simulink model "Yaw_Diff_CS9_Lab"  (R2020a)
settings: Solver=ode45  StartTime=0  StopTime=10  FixedStep=0.002  RelTol=1e-3  AbsTol=1e-6
libraries: simulink x4, simulink_extras x2, Solver_SF x1
settings Model: ExtModeTrigMode=oneshot  ExtModeArmWhenConnect=off  Creator=ywata  LastModifiedBy=S288668
settings SolverCC: AutoScaleAbsTol=off
settings DataIOCC: SaveFormat=Array  SignalLoggingSaveFormat=ModelDataLogs  ReturnWorkspaceOutputs=off  SignalLoggingName=sigsOut
settings OptimizationCC: BooleanDataType=off  ExpressionDepthLimit=2147483647  LifeSpan=inf
settings DebuggingCC: SaveWithParameterizedLinksMsg=none  UnderspecifiedInitializationDetection=Classic  MergeDetectMultiDrivingBlocksExec=none  SignalResolutionControl=TryResolveAllWithWarning  MultiTaskDSMMsg=warning  MultiTaskCondExecSysMsg=none  FcnCallInpInsideContextMsg=warning  StateNameClashWarn=warning  SFUnexpectedBacktrackingDiag=warning  SFNoUnconditionalDefaultTransitionDiag=warning  SFExecutionAtInitializationDiag=none  ArithmeticOperatorsInVariantConditions=warning
settings HardwareCC: ProdBitPerPointer=32  ProdBitPerSizeT=32  ProdBitPerPtrDiffT=32  ProdLargestAtomicFloat=None  ProdIntDivRoundTo=Undefined  ProdEndianess=Unspecified  ProdWordSize=32  ProdHWDeviceType=32-bit Generic  TargetUnknown=on
settings ModelReferenceCC: PropagateSignalLabelsOutOfModel=off
settings SFSimCC: SimUseLocalCustomCode=off  CustomCodeUndefinedFunction=UseInterfaceOnly
settings RTWCC: TemplateMakefile=grt_vc.tmf  RTWUseLocalCustomCode=off
settings CodeAppCC: StateflowObjectComments=on
settings GRTTargetCC: TargetLangStandard=C89/C90 (ANSI)  CombineOutputUpdateFcns=off  GRTInterface=on
settings ConfigComp: CovMetricSettings=dw  CovHtmlReporting=on  CovSaveCumulativeToWorkspaceVar=on  CovSaveSingleToWorkspaceVar=on  CovExternalEMLEnable=off

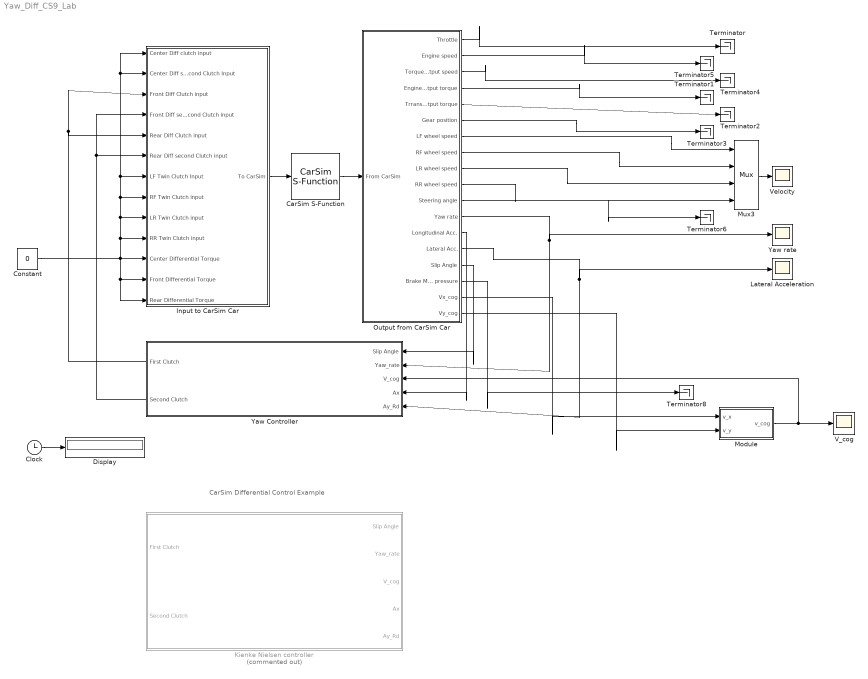
== system Yaw_Diff_CS9_Lab ==
  note: CarSim Differential Control Example
  CarSim S-Function : Solver_SF/CarSim S-Function  Priority=1  SIMFILE=simfile.sim
  Clock : Clock
  Constant : Constant  Value=0
  Display : Display
      settings: Format=bank  Decimation=100
  Input to CarSim Car : Subsystem
  Kienke Nielsen controller : Subsystem  Commented=on
  Lateral Acceleration : Scope
  Module : Subsystem
  Mux3 : Mux
  Output from CarSim Car : Subsystem
  Terminator{,1..6,8} (8 alike) : Terminator
  V_cog : Scope
  Velocity : Scope
  Yaw Controller : Subsystem  mask{YAW=0.06, CONTROL=0.72}
      mask prompts: YAW "Yaw Control Gain (-)"; CONTROL "Control Gain (-)"
  Yaw rate : Scope
  wires:
  Constant/1 -> Input to CarSim Car/11(Center Differential Torque), Input to CarSim Car/12("Front Differential Torque "), Input to CarSim Car/13(Rear Differential Torque), Input to CarSim Car/8(RF Twin Clutch input), Input to CarSim Car/7(LF Twin Clutch Input), Input to CarSim Car/2(Center Diff second Clutch Input), Input to CarSim Car/1(Center Diff clutch input), Input to CarSim Car/9(LR Twin Clutch input), Input to CarSim Car/10(RR Twin Clutch input)
  CarSim S-Function/1 -> Output from CarSim Car/1(From CarSim)
  Input to CarSim Car/1(To CarSim) -> CarSim S-Function/1
  Yaw Controller/1(First Clutch) -> Input to CarSim Car/3(Front Diff Clutch input), Input to CarSim Car/5(Rear Diff Clutch input)
  Yaw Controller/2(Second Clutch) -> Input to CarSim Car/4(Front Diff second Clutch input), Input to CarSim Car/6(Rear Diff second Clutch input)
  Clock/1 -> Display/1
  Mux3/1 -> Velocity/1
  Output from CarSim Car/7(LF wheel speed) -> Mux3/1
  Output from CarSim Car/8(RF wheel speed) -> Mux3/2
  Output from CarSim Car/9(LR wheel speed) -> Mux3/3
  Output from CarSim Car/10(RR wheel speed) -> Mux3/4
  Output from CarSim Car/1(Throttle) -> Terminator/1
  Output from CarSim Car/4(Engine output torque) -> Terminator1/1
  Output from CarSim Car/5(Trransmission output torque) -> Terminator2/1
  Output from CarSim Car/6(Gear position) -> Terminator3/1
  Output from CarSim Car/3(Torque converter output speed) -> Terminator4/1
  Output from CarSim Car/2(Engine speed) -> Terminator5/1
  Output from CarSim Car/11(Steering angle) -> Terminator6/1
  Output from CarSim Car/13(Longitudinal Acc.) -> Yaw Controller/4(Ax)
  Output from CarSim Car/16(Brake M/C pressure) -> Terminator8/1
  Output from CarSim Car/14(Lateral Acc.) -> Yaw Controller/5(Ay_Rd), Lateral Acceleration/1
  Output from CarSim Car/15(Slip Angle) -> Yaw Controller/1(Slip Angle)
  Output from CarSim Car/12(Yaw rate) -> Yaw Controller/2(Yaw_rate), Yaw rate/1
  Output from CarSim Car/17(Vx_cog) -> Module/1(v_x)
  Output from CarSim Car/18(Vy_cog) -> Module/2(v_y)
  Module/1(v_cog) -> V_cog/1, Yaw Controller/3(V_cog)

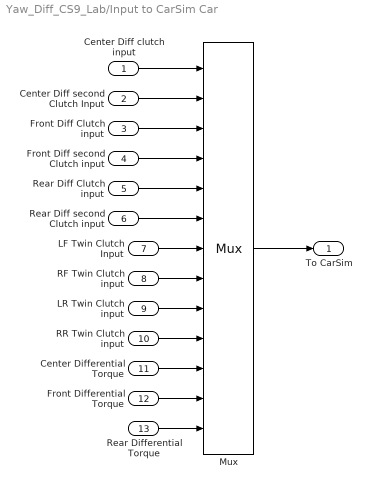
== system Yaw_Diff_CS9_Lab/Input to CarSim Car ==
  Center Diff clutch input : Inport
  Center Diff second Clutch Input : Inport  Port=2
  Front Diff Clutch input : Inport  Port=3
  Front Diff second Clutch input : Inport  Port=4
  Rear Diff Clutch input : Inport  Port=5
  Rear Diff second Clutch input : Inport  Port=6
  LF Twin Clutch Input : Inport  Port=7
  RF Twin Clutch input : Inport  Port=8
  LR Twin Clutch input : Inport  Port=9
  RR Twin Clutch input : Inport  Port=10
  Center Differential Torque : Inport  Port=11
  "Front Differential Torque " : Inport  Port=12
  Rear Differential Torque : Inport  Port=13
  Mux : Mux  Inputs=13
  To CarSim : Outport
  wires:
  Mux/1 -> To CarSim/1
  Center Differential Torque/1 -> Mux/11
  Rear Differential Torque/1 -> Mux/13
  "Front Differential Torque "/1 -> Mux/12
  RR Twin Clutch input/1 -> Mux/10
  LR Twin Clutch input/1 -> Mux/9
  RF Twin Clutch input/1 -> Mux/8
  LF Twin Clutch Input/1 -> Mux/7
  Rear Diff second Clutch input/1 -> Mux/6
  Rear Diff Clutch input/1 -> Mux/5
  Front Diff second Clutch input/1 -> Mux/4
  Front Diff Clutch input/1 -> Mux/3
  Center Diff second Clutch Input/1 -> Mux/2
  Center Diff clutch input/1 -> Mux/1

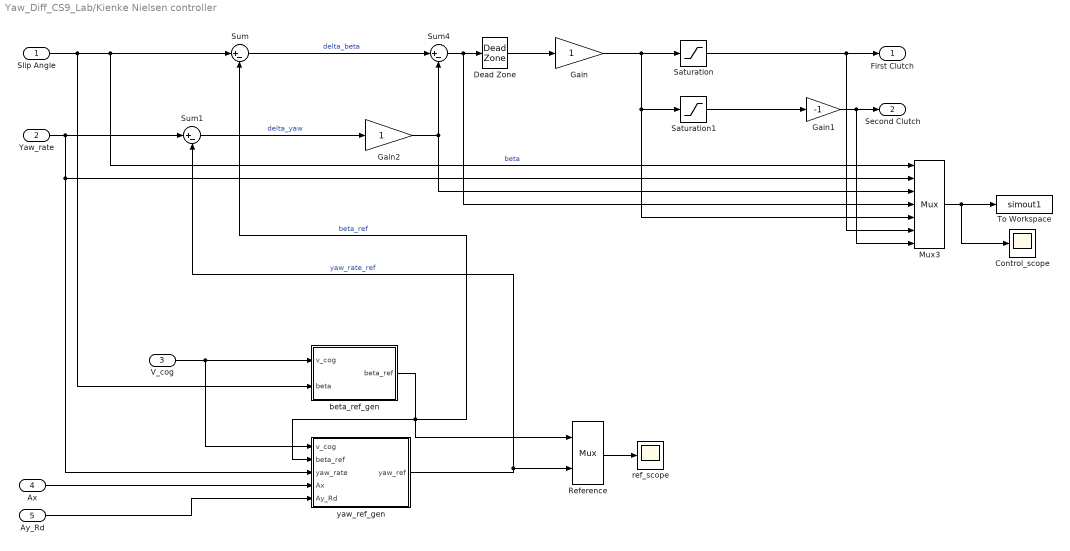
== system Yaw_Diff_CS9_Lab/Kienke Nielsen controller ==
  Slip Angle : Inport
  Yaw_rate : Inport  Port=2
  V_cog : Inport  Port=3
  Ax : Inport  Port=4
  Ay_Rd : Inport  Port=5
  Control_scope : Scope
  Dead Zone : DeadZone  SaturateOnIntegerOverflow=on
  Gain : Gain
  Gain1 : Gain  Gain=-1  SaturateOnIntegerOverflow=on  OutDataTypeStr=Inherit: Same as input  ParamDataTypeStr=Inherit: Same as input
  Gain2 : Gain
  Mux3 : Mux  Inputs=7
  Reference : Mux  Inputs=2
  Saturation : Saturate  UpperLimit=1  LowerLimit=0
  Saturation1 : Saturate  UpperLimit=0  LowerLimit=-1
  Sum : Sum  Inputs=|+-
  Sum1 : Sum  Inputs=|+-
  Sum4 : Sum  Inputs=|+-  InputSameDT=on  SaturateOnIntegerOverflow=on  OutDataTypeStr=Inherit: Same as first input
  To Workspace : ToWorkspace  VariableName=simout1  SaveFormat=Timeseries  SampleTime=-1
  beta_ref_gen : Subsystem
  ref_scope : Scope
  yaw_ref_gen : Subsystem
  First Clutch : Outport
  Second Clutch : Outport  Port=2
  wires:
  yaw_ref_gen/1(yaw_ref) -> Sum1/2, Reference/2  "yaw_rate_ref"
  Ay_Rd/1 -> yaw_ref_gen/5(Ay_Rd)
  Gain1/1 -> Mux3/7, Second Clutch/1
  Mux3/1 -> To Workspace/1, Control_scope/1
  V_cog/1 -> yaw_ref_gen/1(v_cog), beta_ref_gen/1(v_cog)
  Saturation/1 -> Mux3/6, First Clutch/1
  beta_ref_gen/1(beta_ref) -> yaw_ref_gen/2(beta_ref), Sum/2, Reference/1  "beta_ref"
  Slip Angle/1 -> Sum/1, Mux3/1, beta_ref_gen/2(beta)  "beta"
  Sum4/1 -> Mux3/4, Dead Zone/1
  Reference/1 -> ref_scope/1
  Ax/1 -> yaw_ref_gen/4(Ax)
  Yaw_rate/1 -> Sum1/1, yaw_ref_gen/3(yaw_rate), Mux3/2
  Saturation1/1 -> Gain1/1
  Gain/1 -> Saturation/1, Mux3/5, Saturation1/1
  Dead Zone/1 -> Gain/1
  Gain2/1 -> Mux3/3, Sum4/2
  Sum/1 -> Sum4/1  "delta_beta"
  Sum1/1 -> Gain2/1  "delta_yaw"

== system Yaw_Diff_CS9_Lab/Module ==
  v_x : Inport
  v_y : Inport  Port=2
  Sqrt : Sqrt  SaturateOnIntegerOverflow=on
  Square : Math  Operator=square  SaturateOnIntegerOverflow=on
  Square1 : Math  Operator=square  SaturateOnIntegerOverflow=on
  Sum : Sum  Inputs=|++
  v_cog : Outport
  wires:
  v_x/1 -> Square/1
  v_y/1 -> Square1/1
  Square/1 -> Sum/1
  Square1/1 -> Sum/2
  Sum/1 -> Sqrt/1
  Sqrt/1 -> v_cog/1

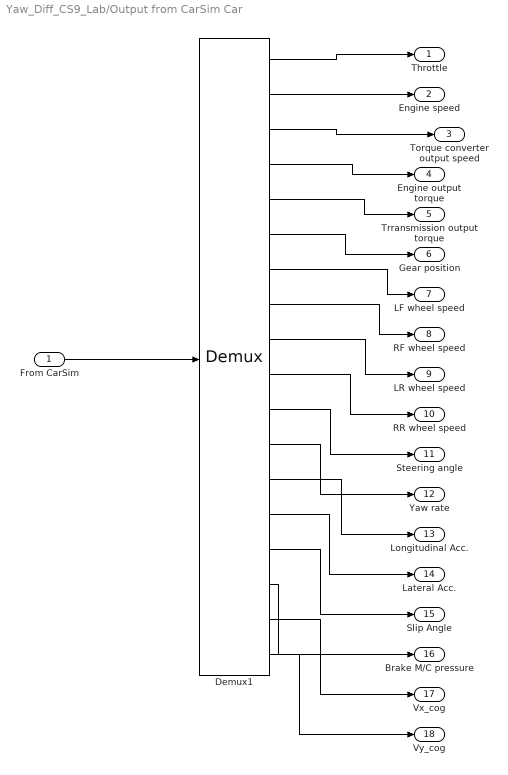
== system Yaw_Diff_CS9_Lab/Output from CarSim Car ==
  From CarSim : Inport
  Demux1 : Demux  Outputs=18
      settings: DisplayOption=none
  Throttle : Outport
  Engine speed : Outport  Port=2
  Torque converter output speed : Outport  Port=3
  Engine output torque : Outport  Port=4
  Trransmission output torque : Outport  Port=5
  Gear position : Outport  Port=6
  LF wheel speed : Outport  Port=7
  RF wheel speed : Outport  Port=8
  LR wheel speed : Outport  Port=9
  RR wheel speed : Outport  Port=10
  Steering angle : Outport  Port=11
  Yaw rate : Outport  Port=12
  Longitudinal Acc. : Outport  Port=13
  Lateral Acc. : Outport  Port=14
  Slip Angle : Outport  Port=15
  Brake M/C pressure : Outport  Port=16
  Vx_cog : Outport  Port=17
  Vy_cog : Outport  Port=18
  wires:
  From CarSim/1 -> Demux1/1
  Demux1/1 -> Throttle/1
  Demux1/2 -> Engine speed/1
  Demux1/3 -> Torque converter output speed/1
  Demux1/7 -> LF wheel speed/1
  Demux1/13 -> Longitudinal Acc./1
  Demux1/14 -> Lateral Acc./1
  Demux1/8 -> RF wheel speed/1
  Demux1/9 -> LR wheel speed/1
  Demux1/10 -> RR wheel speed/1
  Demux1/11 -> Steering angle/1
  Demux1/12 -> Yaw rate/1
  Demux1/4 -> Engine output torque/1
  Demux1/5 -> Trransmission output torque/1
  Demux1/6 -> Gear position/1
  Demux1/15 -> Slip Angle/1
  Demux1/16 -> Brake M/C pressure/1
  Demux1/17 -> Vx_cog/1
  Demux1/18 -> Vy_cog/1

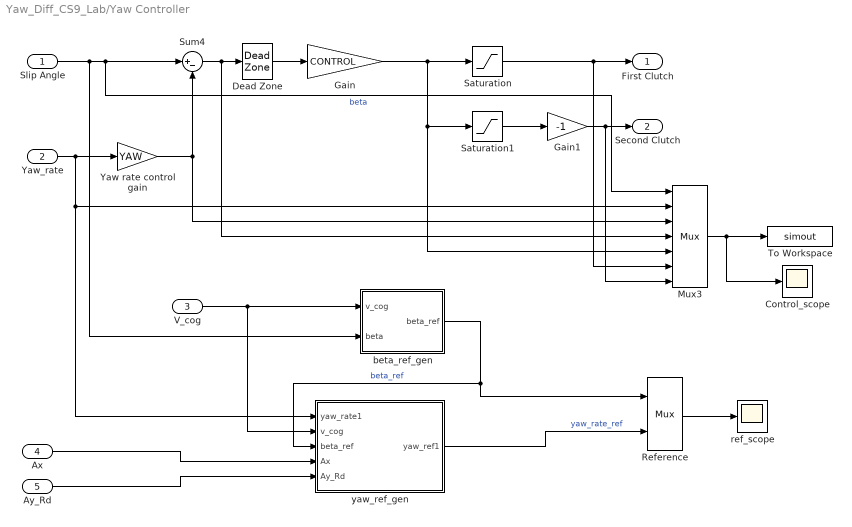
== system Yaw_Diff_CS9_Lab/Yaw Controller ==
  Slip Angle : Inport
  Yaw_rate : Inport  Port=2
  V_cog : Inport  Port=3
  Ax : Inport  Port=4
  Ay_Rd : Inport  Port=5
  Control_scope : Scope
  Dead Zone : DeadZone  SaturateOnIntegerOverflow=on
  Gain : Gain  Gain=CONTROL  SaturateOnIntegerOverflow=on  OutDataTypeStr=Inherit: Same as input  ParamDataTypeStr=Inherit: Same as input
  Gain1 : Gain  Gain=-1  SaturateOnIntegerOverflow=on  OutDataTypeStr=Inherit: Same as input  ParamDataTypeStr=Inherit: Same as input
  Mux3 : Mux  Inputs=7
  Reference : Mux  Inputs=2
  Saturation : Saturate  UpperLimit=1  LowerLimit=0
  Saturation1 : Saturate  UpperLimit=0  LowerLimit=-1
  Sum4 : Sum  Inputs=|+-  InputSameDT=on  SaturateOnIntegerOverflow=on  OutDataTypeStr=Inherit: Same as first input
  To Workspace : ToWorkspace  VariableName=simout  SaveFormat=Timeseries  SampleTime=-1
  Yaw rate control gain : Gain  Gain=YAW  SaturateOnIntegerOverflow=on  OutDataTypeStr=Inherit: Same as input  ParamDataTypeStr=Inherit: Same as input
  beta_ref_gen : Subsystem
  ref_scope : Scope
  yaw_ref_gen : Subsystem
  First Clutch : Outport
  Second Clutch : Outport  Port=2
  wires:
  Yaw rate control gain/1 -> Mux3/3, Sum4/2
  Yaw_rate/1 -> yaw_ref_gen/1(yaw_rate1), Mux3/2, Yaw rate control gain/1
  Dead Zone/1 -> Gain/1
  Sum4/1 -> Mux3/4, Dead Zone/1
  Gain/1 -> Saturation/1, Mux3/5, Saturation1/1
  Saturation1/1 -> Gain1/1
  Saturation/1 -> Mux3/6, First Clutch/1
  Gain1/1 -> Mux3/7, Second Clutch/1
  Slip Angle/1 -> Mux3/1, Sum4/1, beta_ref_gen/2(beta)  "beta"
  Mux3/1 -> To Workspace/1, Control_scope/1
  Reference/1 -> ref_scope/1
  V_cog/1 -> yaw_ref_gen/2(v_cog), beta_ref_gen/1(v_cog)
  beta_ref_gen/1(beta_ref) -> yaw_ref_gen/3(beta_ref), Reference/1  "beta_ref"
  yaw_ref_gen/1(yaw_ref1) -> Reference/2  "yaw_rate_ref"
  Ay_Rd/1 -> yaw_ref_gen/5(Ay_Rd)
  Ax/1 -> yaw_ref_gen/4(Ax)

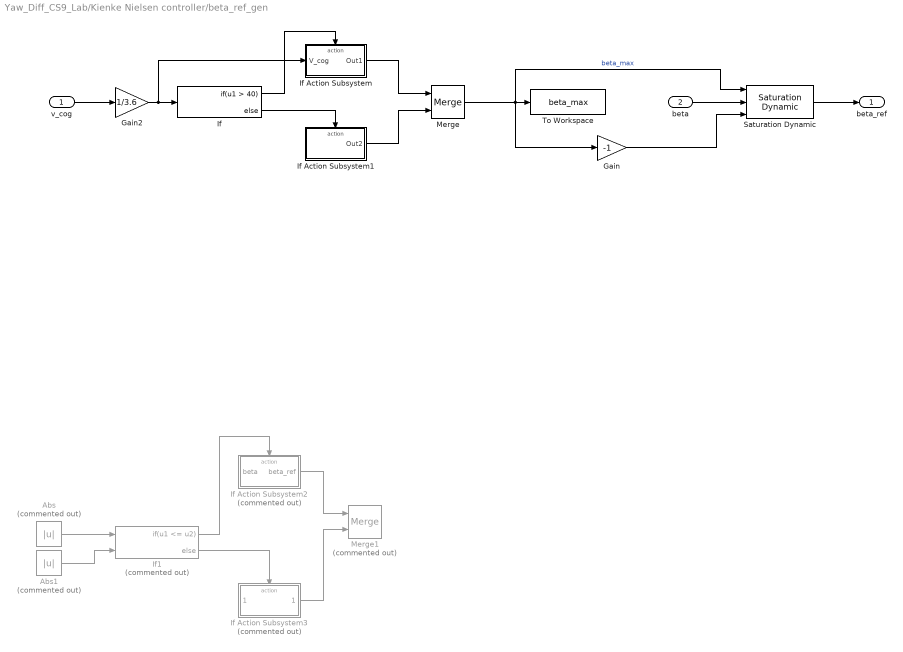
== system Yaw_Diff_CS9_Lab/Kienke Nielsen controller/beta_ref_gen ==
  v_cog : Inport
  beta : Inport  Port=2
  Abs : Abs  Commented=on
  Abs1 : Abs  Commented=on
  Gain : Gain  Gain=-1
  Gain2 : Gain  Gain=1/3.6
  If : If  IfExpression=u1 > 40
  If Action Subsystem : Subsystem  TreatAsAtomicUnit=on
  If Action Subsystem1 : Subsystem  TreatAsAtomicUnit=on
  If Action Subsystem2 : Subsystem  Commented=on  TreatAsAtomicUnit=on
  If Action Subsystem3 : Subsystem  Commented=on  TreatAsAtomicUnit=on
  If1 : If  Commented=on  NumInputs=2  IfExpression=u1 <= u2
  Merge : Merge
  Merge1 : Merge  Commented=on
  Saturation Dynamic : simulink/Discontinuities/Saturation Dynamic  OutMin=[]  OutMax=[]  OutDataTypeStr=Inherit: Same as second input  OutDataType=fixdt(1, 16)  OutScaling=2^-10  DoSatur=off
  To Workspace : ToWorkspace  VariableName=beta_max  SaveFormat=Timeseries  SampleTime=-1
  beta_ref : Outport
  wires:
  If/1 -> If Action Subsystem/Action
  Gain2/1 -> If Action Subsystem/1(V_cog), If/1
  If Action Subsystem/1(Out1) -> Merge/1
  If/2 -> If Action Subsystem1/Action
  If Action Subsystem1/1(Out2) -> Merge/2
  v_cog/1 -> Gain2/1
  Merge/1 -> Gain/1, Saturation Dynamic/1, To Workspace/1  "beta_max"
  Abs1/1 -> If1/2
  ? -> If Action Subsystem2/1(beta), Abs/1
  If1/2 -> If Action Subsystem3/Action
  Abs/1 -> If1/1
  If Action Subsystem3/1(beta_ref) -> Merge1/2
  If Action Subsystem2/1(beta_ref) -> Merge1/1
  ? -> If Action Subsystem3/1(beta_max), Abs1/1  "beta_max"
  If1/1 -> If Action Subsystem2/Action
  Saturation Dynamic/1 -> beta_ref/1
  beta/1 -> Saturation Dynamic/2
  Gain/1 -> Saturation Dynamic/3

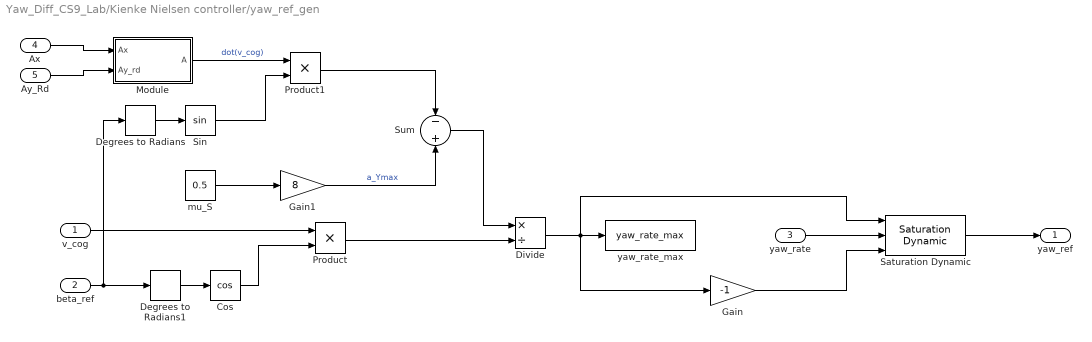
== system Yaw_Diff_CS9_Lab/Kienke Nielsen controller/yaw_ref_gen ==
  v_cog : Inport
  beta_ref : Inport  Port=2
  yaw_rate : Inport  Port=3
  Ax : Inport  Port=4
  Ay_Rd : Inport  Port=5
  Cos : Trigonometry  Operator=cos
  Degrees to Radians : simulink_extras/Transformations/Degrees to Radians
  Degrees to Radians1 : simulink_extras/Transformations/Degrees to Radians
  Divide : Product  Inputs=*/
  Gain : Gain  Gain=-1
  Gain1 : Gain  Gain=8
  Module : Subsystem
  Product : Product
  Product1 : Product
  Saturation Dynamic : simulink/Discontinuities/Saturation Dynamic  OutMin=[]  OutMax=[]  OutDataTypeStr=Inherit: Same as second input  OutDataType=fixdt(1, 16)  OutScaling=2^-10  DoSatur=off
  Sin : Trigonometry
  Sum : Sum  Inputs=-|+
  mu_S : Constant  Value=0.5
  yaw_rate_max : ToWorkspace  VariableName=yaw_rate_max  SaveFormat=Timeseries  SampleTime=-1
  yaw_ref : Outport
  wires:
  beta_ref/1 -> Degrees to Radians/1, Degrees to Radians1/1
  v_cog/1 -> Product/1
  Cos/1 -> Product/2
  Sin/1 -> Product1/2
  Product1/1 -> Sum/1
  Product/1 -> Divide/2
  Sum/1 -> Divide/1
  Divide/1 -> Gain/1, Saturation Dynamic/1, yaw_rate_max/1
  yaw_rate/1 -> Saturation Dynamic/2
  Saturation Dynamic/1 -> yaw_ref/1
  Module/1(A) -> Product1/1  "dot(v_cog)"
  Ax/1 -> Module/1(Ax)
  Ay_Rd/1 -> Module/2(Ay_rd)
  mu_S/1 -> Gain1/1
  Gain1/1 -> Sum/2  "a_Ymax"
  Gain/1 -> Saturation Dynamic/3
  Degrees to Radians/1 -> Sin/1
  Degrees to Radians1/1 -> Cos/1

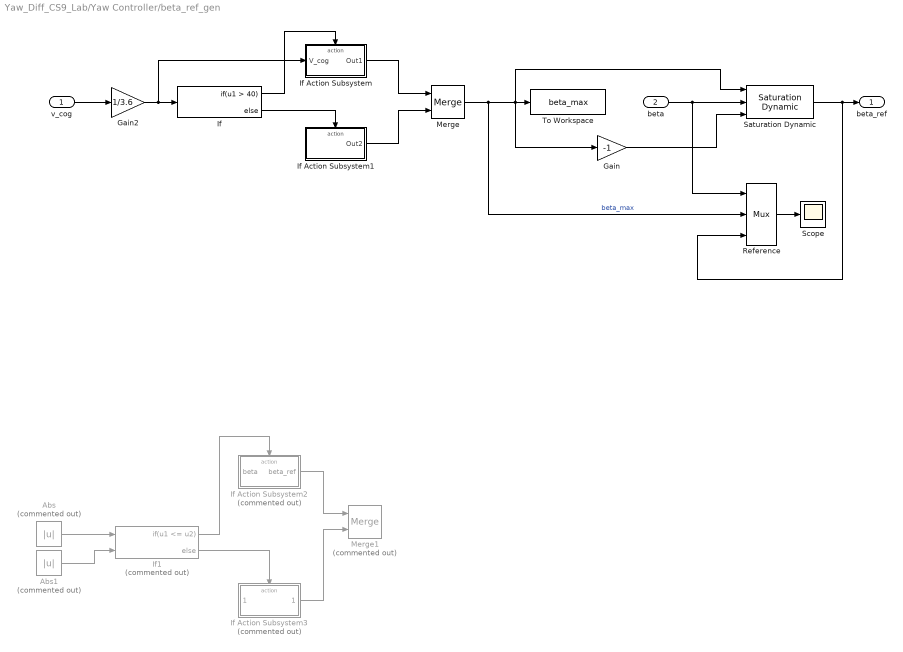
== system Yaw_Diff_CS9_Lab/Yaw Controller/beta_ref_gen ==
  v_cog : Inport
  beta : Inport  Port=2
  Abs : Abs  Commented=on
  Abs1 : Abs  Commented=on
  Gain : Gain  Gain=-1
  Gain2 : Gain  Gain=1/3.6
  If : If  IfExpression=u1 > 40
  If Action Subsystem : Subsystem  TreatAsAtomicUnit=on
  If Action Subsystem1 : Subsystem  TreatAsAtomicUnit=on
  If Action Subsystem2 : Subsystem  Commented=on  TreatAsAtomicUnit=on
  If Action Subsystem3 : Subsystem  Commented=on  TreatAsAtomicUnit=on
  If1 : If  Commented=on  NumInputs=2  IfExpression=u1 <= u2
  Merge : Merge
  Merge1 : Merge  Commented=on
  Reference : Mux  Inputs=3
  Saturation Dynamic : simulink/Discontinuities/Saturation Dynamic  OutMin=[]  OutMax=[]  OutDataTypeStr=Inherit: Same as second input  OutDataType=fixdt(1, 16)  OutScaling=2^-10  DoSatur=off
  Scope : Scope
  To Workspace : ToWorkspace  VariableName=beta_max  SaveFormat=Timeseries  SampleTime=-1
  beta_ref : Outport
  wires:
  If/1 -> If Action Subsystem/Action
  Gain2/1 -> If Action Subsystem/1(V_cog), If/1
  If Action Subsystem/1(Out1) -> Merge/1
  If/2 -> If Action Subsystem1/Action
  If Action Subsystem1/1(Out2) -> Merge/2
  v_cog/1 -> Gain2/1
  Merge/1 -> Reference/2, Gain/1, Saturation Dynamic/1, To Workspace/1  "beta_max"
  Abs1/1 -> If1/2
  ? -> If Action Subsystem2/1(beta), Abs/1
  If1/2 -> If Action Subsystem3/Action
  Abs/1 -> If1/1
  If Action Subsystem3/1(beta_ref) -> Merge1/2
  If Action Subsystem2/1(beta_ref) -> Merge1/1
  ? -> If Action Subsystem3/1(beta_max), Abs1/1  "beta_max"
  If1/1 -> If Action Subsystem2/Action
  Saturation Dynamic/1 -> Reference/3, beta_ref/1
  beta/1 -> Reference/1, Saturation Dynamic/2
  Gain/1 -> Saturation Dynamic/3
  Reference/1 -> Scope/1

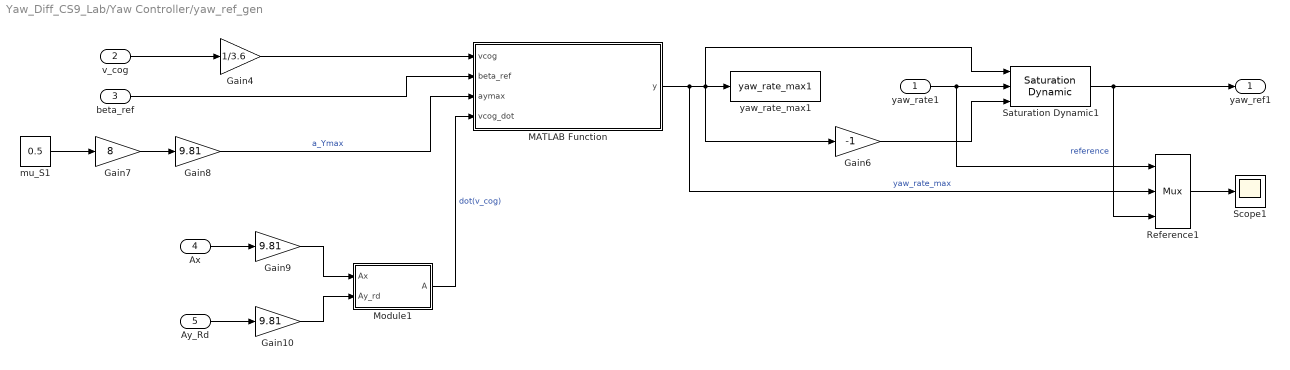
== system Yaw_Diff_CS9_Lab/Yaw Controller/yaw_ref_gen ==
  yaw_rate1 : Inport
  v_cog : Inport  Port=2
  beta_ref : Inport  Port=3
  Ax : Inport  Port=4
  Ay_Rd : Inport  Port=5
  Gain10 : Gain  Gain=9.81
  Gain4 : Gain  Gain=1/3.6
  Gain6 : Gain  Gain=-1
  Gain7 : Gain  Gain=8
  Gain8 : Gain  Gain=9.81
  Gain9 : Gain  Gain=9.81
  MATLAB Function : MATLAB Function  TreatAsAtomicUnit=on
  Module1 : Subsystem
  Reference1 : Mux  Inputs=3
  Saturation Dynamic1 : simulink/Discontinuities/Saturation Dynamic  OutMin=[]  OutMax=[]  OutDataTypeStr=Inherit: Same as second input  OutDataType=fixdt(1, 16)  OutScaling=2^-10  DoSatur=off
  Scope1 : Scope
  mu_S1 : Constant  Value=0.5
  yaw_rate_max1 : ToWorkspace  VariableName=yaw_rate_max1  SaveFormat=Timeseries  SampleTime=-1
  yaw_ref1 : Outport
  wires:
  Gain6/1 -> Saturation Dynamic1/3
  Saturation Dynamic1/1 -> yaw_ref1/1, Reference1/3  "reference"
  MATLAB Function/1(y) -> Reference1/2, Gain6/1, Saturation Dynamic1/1, yaw_rate_max1/1  "yaw_rate_max"
  yaw_rate1/1 -> Reference1/1, Saturation Dynamic1/2
  Reference1/1 -> Scope1/1
  Gain7/1 -> Gain8/1
  mu_S1/1 -> Gain7/1
  Gain8/1 -> MATLAB Function/3(aymax)  "a_Ymax"
  Gain9/1 -> Module1/1(Ax)
  Module1/1(A) -> MATLAB Function/4(vcog_dot)  "dot(v_cog)"
  Gain10/1 -> Module1/2(Ay_rd)
  v_cog/1 -> Gain4/1
  Gain4/1 -> MATLAB Function/1(vcog)
  beta_ref/1 -> MATLAB Function/2(beta_ref)
  Ay_Rd/1 -> Gain10/1
  Ax/1 -> Gain9/1

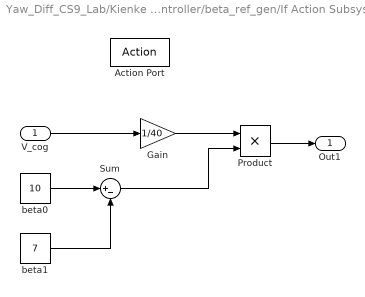
== system Yaw_Diff_CS9_Lab/Kienke Nielsen controller/beta_ref_gen/If Action Subsystem ==
  V_cog : Inport
  Action Port : ActionPort
  Gain : Gain  Gain=1/40
  Product : Product
  Sum : Sum  Inputs=|+-
  beta0 : Constant  Value=10
  beta1 : Constant  Value=7
  Out1 : Outport
  wires:
  Sum/1 -> Product/2
  beta0/1 -> Sum/1
  Gain/1 -> Product/1
  V_cog/1 -> Gain/1
  Product/1 -> Out1/1
  beta1/1 -> Sum/2

== system Yaw_Diff_CS9_Lab/Kienke Nielsen controller/beta_ref_gen/If Action Subsystem1 ==
  Action Port : ActionPort
  Sum : Sum  Inputs=|+-
  beta0 : Constant  Value=10
  beta1 : Constant  Value=7
  Out2 : Outport
  wires:
  beta0/1 -> Sum/1
  beta1/1 -> Sum/2
  Sum/1 -> Out2/1

== system Yaw_Diff_CS9_Lab/Kienke Nielsen controller/beta_ref_gen/If Action Subsystem2 ==
  beta : Inport
  Action Port : ActionPort
  beta_ref : Outport
  wires:
  beta/1 -> beta_ref/1

== system Yaw_Diff_CS9_Lab/Kienke Nielsen controller/beta_ref_gen/If Action Subsystem3 ==
  beta_max : Inport
  Action Port : ActionPort
  beta_ref : Outport
  wires:
  beta_max/1 -> beta_ref/1

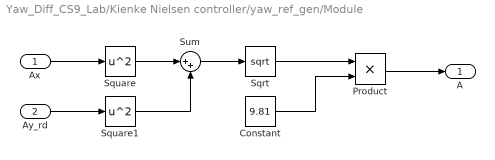
== system Yaw_Diff_CS9_Lab/Kienke Nielsen controller/yaw_ref_gen/Module ==
  Ax : Inport
  Ay_rd : Inport  Port=2
  Constant : Constant  Value=9.81
  Product : Product
  Sqrt : Sqrt  SaturateOnIntegerOverflow=on
  Square : Math  Operator=square  SaturateOnIntegerOverflow=on
  Square1 : Math  Operator=square  SaturateOnIntegerOverflow=on
  Sum : Sum  Inputs=|++
  A : Outport
  wires:
  Ax/1 -> Square/1
  Ay_rd/1 -> Square1/1
  Constant/1 -> Product/2
  Sqrt/1 -> Product/1
  Square/1 -> Sum/1
  Square1/1 -> Sum/2
  Sum/1 -> Sqrt/1
  Product/1 -> A/1

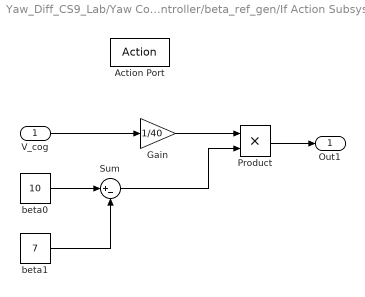
== system Yaw_Diff_CS9_Lab/Yaw Controller/beta_ref_gen/If Action Subsystem ==
  V_cog : Inport
  Action Port : ActionPort  ActionPortLabel=if(u1 > 40)
  Gain : Gain  Gain=1/40
  Product : Product
  Sum : Sum  Inputs=|+-
  beta0 : Constant  Value=10
  beta1 : Constant  Value=7
  Out1 : Outport
  wires:
  Sum/1 -> Product/2
  beta0/1 -> Sum/1
  Gain/1 -> Product/1
  V_cog/1 -> Gain/1
  Product/1 -> Out1/1
  beta1/1 -> Sum/2

== system Yaw_Diff_CS9_Lab/Yaw Controller/beta_ref_gen/If Action Subsystem1 ==
  Action Port : ActionPort  ActionPortLabel=else
  Sum : Sum  Inputs=|+-
  beta0 : Constant  Value=10
  beta1 : Constant  Value=7
  Out2 : Outport
  wires:
  beta0/1 -> Sum/1
  beta1/1 -> Sum/2
  Sum/1 -> Out2/1

== system Yaw_Diff_CS9_Lab/Yaw Controller/beta_ref_gen/If Action Subsystem2 ==
  beta : Inport
  Action Port : ActionPort  ActionPortLabel=if(u1 <= u2)
  beta_ref : Outport
  wires:
  beta/1 -> beta_ref/1

== system Yaw_Diff_CS9_Lab/Yaw Controller/beta_ref_gen/If Action Subsystem3 ==
  beta_max : Inport
  Action Port : ActionPort  ActionPortLabel=else
  beta_ref : Outport
  wires:
  beta_max/1 -> beta_ref/1

== system Yaw_Diff_CS9_Lab/Yaw Controller/yaw_ref_gen/Module1 ==
  Ax : Inport
  Ay_rd : Inport  Port=2
  Sqrt : Sqrt  SaturateOnIntegerOverflow=on
  Square : Math  Operator=square  SaturateOnIntegerOverflow=on
  Square1 : Math  Operator=square  SaturateOnIntegerOverflow=on
  Sum : Sum  Inputs=|++
  A : Outport
  wires:
  Ax/1 -> Square/1
  Ay_rd/1 -> Square1/1
  Square/1 -> Sum/1
  Square1/1 -> Sum/2
  Sum/1 -> Sqrt/1
  Sqrt/1 -> A/1

== matlab function Yaw_Diff_CS9_Lab/Yaw Controller/yaw_ref_gen/MATLAB Function ==
  data: vcog input; y output; beta_ref input; aymax input; vcog_dot input
function y = yawmax(vcog,beta_ref,aymax,vcog_dot)
beta_ref = deg2rad(beta_ref);
y = 1/(vcog*cos(beta_ref))*(aymax - vcog_dot*sin(beta_ref));
